simulink model "simulateur_pendule"  (R2023a)
settings: Solver=VariableStepAuto  StartTime=0.0  StopTime=5  RelTol=1e-3
values from neighbouring files (symbols this model uses):
  K = place(A,B,polesoute)    [test.m]
settings Model: Creator=Morin  LastModifiedBy=haoyuan
settings SolverCC: AlgebraicLoopSolver=TrustRegion
settings DebuggingCC: UnconnectedInputMsg=warning  UnconnectedOutputMsg=warning  UnconnectedLineMsg=warning
settings ModelReferenceCC: EnableRefExpFcnMdlSchedulingChecks=on

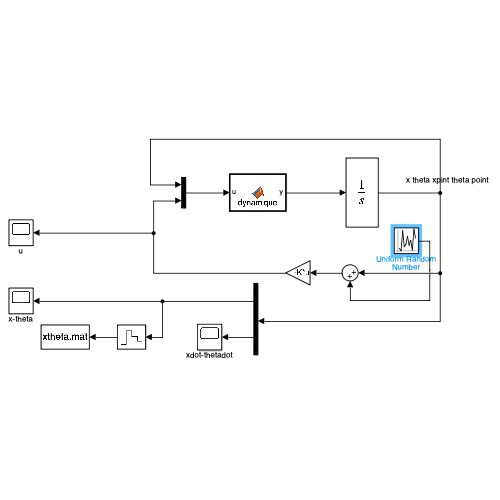
[thumbnail: Simulink's stored preview of the top-level diagram]
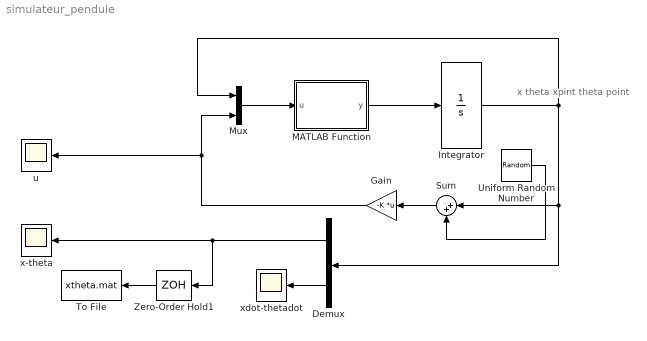
== system simulateur_pendule ==
  note: x theta xpint theta point
  Demux : Demux  Outputs=2
  Gain : Gain  Gain=-K  Multiplication=Matrix(K*u)
  Integrator : Integrator  InitialCondition=[0;0.3;0;0]
  MATLAB Function : MATLAB Function  TreatAsAtomicUnit=on
  Mux : Mux  Inputs=2
  Sum : Sum  Inputs=|++
  To File : ToFile  Filename=xtheta.mat  SaveFormat=Timeseries  SampleTime=0.01
  Uniform Random Number : UniformRandomNumber  Minimum=-0.02  Maximum=0.02  SampleTime=1/1000
  Zero-Order Hold1 : ZeroOrderHold  SampleTime=0.01
  u : Scope
  x-theta : Scope
  xdot-thetadot : Scope
  wires:
  MATLAB Function/1(y) -> Integrator/1
  Integrator/1 -> Mux/1, Sum/1, Demux/1
  Mux/1 -> MATLAB Function/1(u)
  Demux/1 -> Zero-Order Hold1/1, x-theta/1
  Demux/2 -> xdot-thetadot/1
  Gain/1 -> u/1, Mux/2
  Zero-Order Hold1/1 -> To File/1
  Sum/1 -> Gain/1
  Uniform Random Number/1 -> Sum/2

== matlab function simulateur_pendule/MATLAB Function ==
  data: u input; y output
function y = dynamique(u)
% fonction définissant la dynamique du système: renvoie f(X,U) avec X
% l'état, et U la variable de commande physique (composante T de la force
% appliquée au chariot)

x= u(1); %position du chariot
theta= u(2); %inclinaison de la barre
xdot= u(3); % vitesse du chariot
thetadot= u(4); % vitesse angulaire de la barre
T= u(5); % force appliquée au chariot

% Defintion des paramètres du système
m= 0.2; % masse de la barre
M= 1; % masse totale (chariot + barre)
l= 0.2 % demi-longueur de la barre
J=  m*l^2/3; % inertie de la barre
g= 9.81; % cste de gravité
mu= 0.005; % coeff. de frottement visqueux barre
tau= 0.2; % coeff. de frottement visqueux chariot

% Calcul des dérivées secondes
Delta_theta= M*(J+m*l^2)-m^2*l^2*(cos(theta))^2;
disp(Delta_theta);
%2*2 2*1
xthetaddot=1/Delta_theta*[J+m*l^2 -m*l*cos(theta);-m*l*cos(theta) M]*...
    [T+m*l*thetadot^2*sin(theta)-tau*xdot;m*g*l*sin(theta)-mu*thetadot];
%Calcul de f
y = [xdot;thetadot;xthetaddot];
